simulink model "dynamicFIRv1"  (R2019b)
settings: Solver=FixedStepAuto  StartTime=0.0  StopTime=stop_time  RelTol=1e-3
InitFcn:
  | init;
StopFcn:
  | output;
values from neighbouring files (symbols this model uses):
  ram_size = 4    [init.m]
  Ts_system = 1/Fs_system    (= 2e-08)    [init.m]
libraries: dsphdlfiltering x1, hdlsllib x1
settings Model: Creator=Showi  LastModifiedBy=Showi

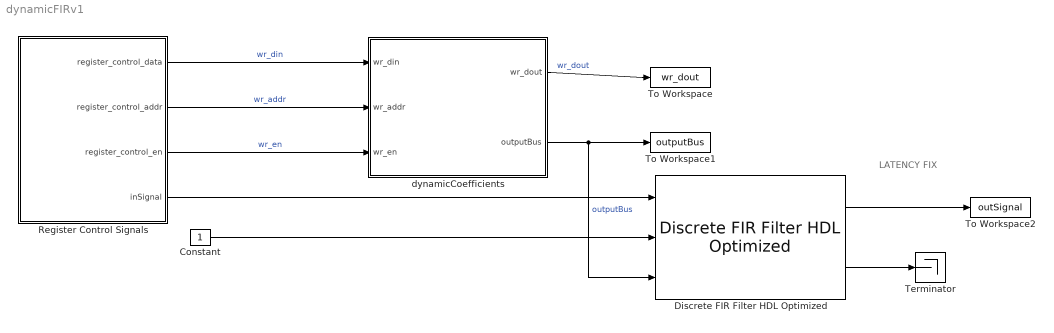
== system dynamicFIRv1 ==
  note: LATENCY FIX
  Constant : Constant  OutDataTypeStr=boolean  SampleTime=-1
  Discrete FIR Filter HDL Optimized : dsphdlfiltering/Discrete FIR Filter HDL Optimized  NumeratorSource=Input port (Parallel interface)  Numerator=[ 0.5, 0.5 ]  NumeratorPrototype=[]  FilterStructure=Direct form systolic  SerializationOption=Minimum number of cycles between valid input samples  NumberOfCycles=2  NumberOfMultipliers=2  SimulateUsing=Code generation  roundingMode=Floor  overflowMode=off  CoefficientsDataTypeStr=Inherit: Same word length as input  CoefficientsMin=[]  CoefficientsMax=[]  OutputMin=[]  OutputMax=[]  ResetInputPort=off  HDLGlobalReset=off
      settings: SourceProductName=DSP System Toolbox  SourceProductBaseCode=DS
  Register Control Signals : Subsystem
  Terminator : Terminator
  To Workspace : ToWorkspace  VariableName=wr_dout  SaveFormat=Timeseries  SampleTime=-1
  To Workspace1 : ToWorkspace  VariableName=outputBus  SaveFormat=Timeseries  SampleTime=-1
  To Workspace2 : ToWorkspace  VariableName=outSignal  SaveFormat=Timeseries  SampleTime=-1
  dynamicCoefficients : Subsystem
  wires:
  Register Control Signals/3(register_control_en) -> dynamicCoefficients/3(wr_en)  "wr_en"
  Register Control Signals/2(register_control_addr) -> dynamicCoefficients/2(wr_addr)  "wr_addr"
  Register Control Signals/1(register_control_data) -> dynamicCoefficients/1(wr_din)  "wr_din"
  dynamicCoefficients/1(wr_dout) -> To Workspace/1  "wr_dout"
  dynamicCoefficients/2(outputBus) -> Discrete FIR Filter HDL Optimized/3, To Workspace1/1  "outputBus"
  Constant/1 -> Discrete FIR Filter HDL Optimized/2
  Register Control Signals/4(inSignal) -> Discrete FIR Filter HDL Optimized/1
  Discrete FIR Filter HDL Optimized/2 -> Terminator/1
  Discrete FIR Filter HDL Optimized/1 -> To Workspace2/1

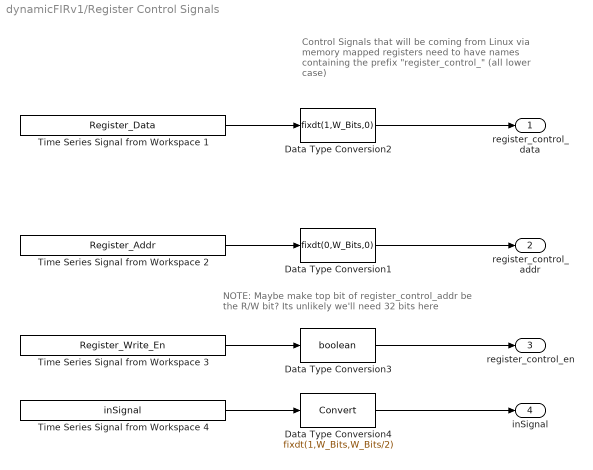
== system dynamicFIRv1/Register Control Signals ==
  note: NOTE: Maybe make top bit of register_control_addr
      | be the R/W bit? Its unlikely we'll need 32 bits here
  note: Control Signals that will be coming from Linux via
      | memory mapped registers need to have names
      | containing the prefix "register_control_"
      | (all lower case)
  Data Type Conversion1 : DataTypeConversion  OutDataTypeStr=fixdt(0,W_Bits,0)
  Data Type Conversion2 : DataTypeConversion  OutDataTypeStr=fixdt(1,W_Bits,0)
  Data Type Conversion3 : DataTypeConversion  OutDataTypeStr=boolean
  Data Type Conversion4 : DataTypeConversion  OutDataTypeStr=fixdt(1,W_Bits,W_Bits/2)
  Time Series Signal from Workspace 1 : FromWorkspace  VariableName=Register_Data  OutDataTypeStr=double  SampleTime=Ts_system  OutputAfterFinalValue=Holding final value
  Time Series Signal from Workspace 2 : FromWorkspace  VariableName=Register_Addr  OutDataTypeStr=double  SampleTime=Ts_system  OutputAfterFinalValue=Holding final value
  Time Series Signal from Workspace 3 : FromWorkspace  VariableName=Register_Write_En  OutDataTypeStr=double  SampleTime=Ts_system  OutputAfterFinalValue=Holding final value
  Time Series Signal from Workspace 4 : FromWorkspace  VariableName=inSignal  OutDataTypeStr=double  SampleTime=Ts_system  OutputAfterFinalValue=Holding final value
  register_control_data : Outport  VectorParamsAs1DForOutWhenUnconnected=off
  register_control_addr : Outport  Port=2  VectorParamsAs1DForOutWhenUnconnected=off
  register_control_en : Outport  Port=3  VectorParamsAs1DForOutWhenUnconnected=off
  inSignal : Outport  Port=4  VectorParamsAs1DForOutWhenUnconnected=off
  wires:
  Time Series Signal from Workspace 1/1 -> Data Type Conversion2/1
  Time Series Signal from Workspace 2/1 -> Data Type Conversion1/1
  Data Type Conversion2/1 -> register_control_data/1
  Data Type Conversion1/1 -> register_control_addr/1
  Time Series Signal from Workspace 3/1 -> Data Type Conversion3/1
  Data Type Conversion3/1 -> register_control_en/1
  Data Type Conversion4/1 -> inSignal/1
  Time Series Signal from Workspace 4/1 -> Data Type Conversion4/1

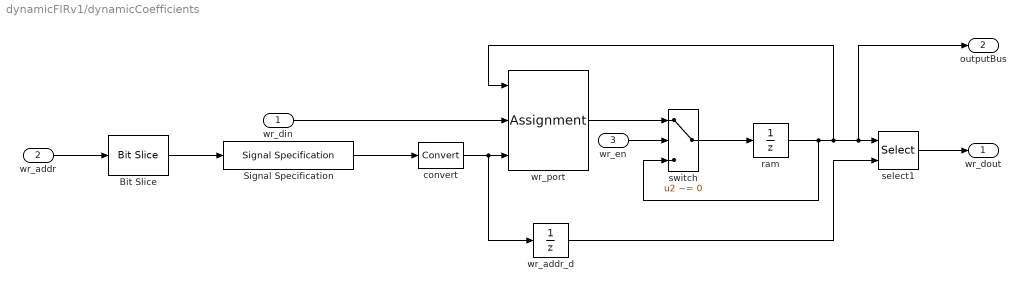
== system dynamicFIRv1/dynamicCoefficients ==
  wr_din : Inport
  wr_addr : Inport  Port=2
  wr_en : Inport  Port=3  OutDataTypeStr=boolean
  Bit Slice : hdlsllib/Logic and Bit Operations/Bit Slice  lidx=ram_size - 1  ridx=0
      settings: SourceProductName=Simulink  SourceProductBaseCode=SL
  Signal Specification : SignalSpecification  OutDataTypeStr=fixdt(0,ram_size,0)  Dimensions=1
  convert : DataTypeConversion
  ram : UnitDelay  SampleTime=-1  HasFrameUpgradeWarning=on
  select1 : Selector  IndexMode=Zero-based  InputPortWidth=2^ram_size  IndexOptions=Index vector (port)  Indices=[1 3]  OutputSizes=1
  switch : Switch  Criteria=u2 ~= 0
  wr_addr_d : UnitDelay  SampleTime=-1  HasFrameUpgradeWarning=on
  wr_port : Assignment  IndexMode=Zero-based  IndexOptions=Index vector (port)  Indices=1  OutputSizes=[1 1]
  wr_dout : Outport  VectorParamsAs1DForOutWhenUnconnected=off
  outputBus : Outport  Port=2  VectorParamsAs1DForOutWhenUnconnected=off
  wires:
  Signal Specification/1 -> convert/1
  wr_addr/1 -> Bit Slice/1
  wr_en/1 -> switch/2
  ram/1 -> wr_port/1, outputBus/1, select1/1, switch/3
  select1/1 -> wr_dout/1
  convert/1 -> wr_port/3, wr_addr_d/1
  switch/1 -> ram/1
  wr_port/1 -> switch/1
  wr_addr_d/1 -> select1/2
  wr_din/1 -> wr_port/2
  Bit Slice/1 -> Signal Specification/1
